simulink model "ex4_model"  (R2024b)
settings: Solver=VariableStepAuto  StartTime=0.0  StopTime=10.0  RelTol=1e-3
values from neighbouring files (symbols this model uses):
  A = [0 1; 0 -20]    [ex_script.m]
  Ao = Ae - Le*Ce    [ex_script.m]
  B = [0; 60]    [ex_script.m]
  Bo = [Be, Le]    [ex_script.m]
  C = [1 0]    [ex_script.m]
  C_r = [1 0 0]    [ex_script.m]
  Co = eye(5, 5)    [ex_script.m]
  D = 0    [ex_script.m]
  Do = zeros(5,2)    [ex_script.m]
  K = place(A_z, B_z, eigs)    [ex_script.m]
  K_e = place (A,B, [p1, conj(p1)])    [ex_script.m]
  sin_w = 6    [ex_script.m]
  w_filt = 2*pi*20    (= 125.663706144)    [ex_script.m]
  zeta_filt = 1/sqrt(2)    [ex_script.m]
settings Model: Creator=Nihal  LastModifiedBy=Nihal

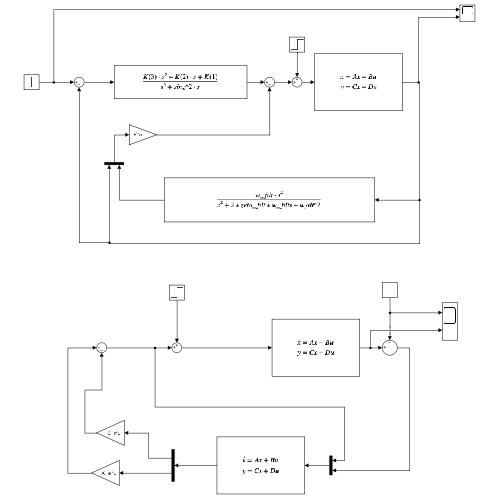
[thumbnail: Simulink's stored preview of the top-level diagram]
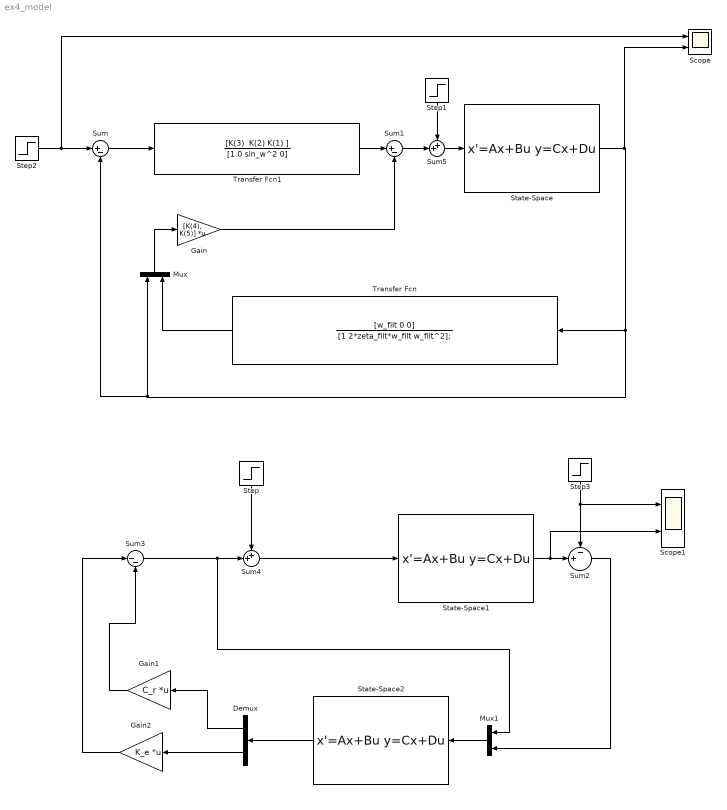
== system ex4_model ==
  Demux : Demux  Outputs=[3,2]
  Gain : Gain  Gain=[K(4), K(5)]  Multiplication=Matrix(K*u)
  Gain1 : Gain  Gain=C_r  Multiplication=Matrix(K*u)
  Gain2 : Gain  Gain=K_e  Multiplication=Matrix(K*u)
  Mux : Mux  Inputs=2
  Mux1 : Mux  Inputs=2
  Scope : Scope  NumInputPorts=2
  Scope1 : Scope  NumInputPorts=2
  State-Space : StateSpace  A=A  B=B  C=C  D=D  InitialCondition=0
  State-Space1 : StateSpace  A=A  B=B  C=C  D=D  InitialCondition=0
  State-Space2 : StateSpace  A=Ao  B=Bo  C=Co  D=Do  InitialCondition=0
  Step{,1..3} (4 alike) : Step  After=50  SampleTime=0
  Sum : Sum  Inputs=|+-
  Sum1 : Sum  Inputs=|+-
  Sum2 : Sum  Inputs=-+|
  Sum3 : Sum  Inputs=|--
  Sum4 : Sum  Inputs=++|
  Sum5 : Sum  Inputs=++|
  Transfer Fcn : TransferFcn  Numerator=[w_filt 0 0]  Denominator=[1 2*zeta_filt*w_filt w_filt^2];
  Transfer Fcn1 : TransferFcn  Numerator="[K(3)  K(2) K(1) ]"  Denominator=[1 0 sin_w^2 0]
  wires:
  State-Space/1 -> Scope/2, Transfer Fcn/1, Sum/2, Mux/1
  Step2/1 -> Scope/1, Sum/1
  Mux/1 -> Gain/1
  Transfer Fcn/1 -> Mux/2
  Sum/1 -> Transfer Fcn1/1
  Transfer Fcn1/1 -> Sum1/1
  Gain/1 -> Sum1/2
  State-Space2/1 -> Demux/1
  State-Space1/1 -> Scope1/2, Sum2/2
  Step3/1 -> Sum2/1, Scope1/1
  Demux/1 -> Gain1/1
  Demux/2 -> Gain2/1
  Gain1/1 -> Sum3/2
  Gain2/1 -> Sum3/1
  Sum3/1 -> Mux1/1, Sum4/2
  Sum4/1 -> State-Space1/1
  Sum2/1 -> Mux1/2
  Mux1/1 -> State-Space2/1
  Sum5/1 -> State-Space/1
  Sum1/1 -> Sum5/2
  Step/1 -> Sum4/1
  Step1/1 -> Sum5/1
